simulink library "LibFactorGraph"  (Simulink 8.3)
settings: Solver=ode45  StartTime=0.0  StopTime=10.0  RelTol=1e-3
undefined symbols (not defined in the file or in its folder): bV, epsVal, eu, fcn, fP_0, fV, Hin_0, L_0, Nit_0, P_0, xi
libraries: LibFactorGraph x357
(part 1 of 4)
settings Model: Creator=amedeobuonanno  LastModifiedBy=amedeo.buonanno

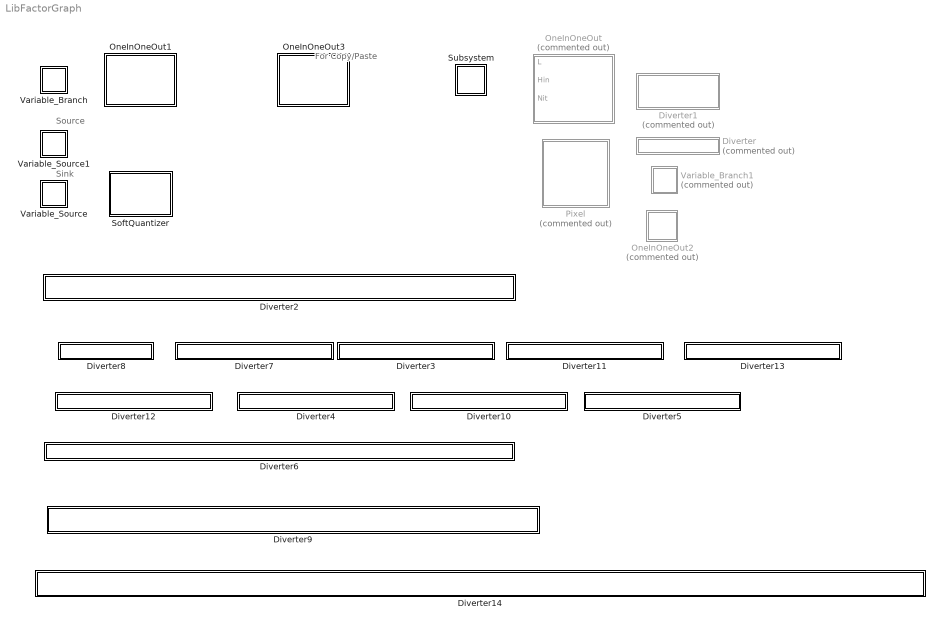
== system LibFactorGraph ==
  note: For Copy/Paste
  note: Source
  note: Sink
  Diverter : Subsystem  Commented=on  mask{up1=up1, up2=up2, down1=down1}
      mask prompts: up1 "Variable Up1"; up2 "Variable Up2"; down1 "Variable Down1"
      mask init:
      | % Set mask modifiable useful?
      | set_param(gcb,'MaskSelfModifiable','on');
      mask Display:
      | %port_label('lconn',1,up1);
      | %port_label('lconn',2,up2);
      | %port_label('rconn',1,down1);
  Diverter1 : Subsystem  Commented=on  mask{up1=up1, up2=up2, down1=down1}
      mask prompts: up1 "Variable Up1"; up2 "Variable Up2"; down1 "Variable Down1"
      mask init:
      | % Set mask modifiable useful?
      | set_param(gcb,'MaskSelfModifiable','on');
      mask Display:
      | port_label('lconn',1,up1);
      | port_label('lconn',2,up2);
      | port_label('rconn',1,down1);
  Diverter10 : Subsystem
      mask init:
      | % Set mask modifiable useful?
      | set_param(gcb,'MaskSelfModifiable','on');
  Diverter11 : Subsystem
      mask init:
      | % Set mask modifiable useful?
      | set_param(gcb,'MaskSelfModifiable','on');
  Diverter12 : Subsystem
      mask init:
      | % Set mask modifiable useful?
      | set_param(gcb,'MaskSelfModifiable','on');
  Diverter13 : Subsystem
      mask init:
      | % Set mask modifiable useful?
      | set_param(gcb,'MaskSelfModifiable','on');
  Diverter14 : Subsystem
      mask init:
      | % Set mask modifiable useful?
      | set_param(gcb,'MaskSelfModifiable','on');
  Diverter2 : Subsystem
      mask init:
      | % Set mask modifiable useful?
      | set_param(gcb,'MaskSelfModifiable','on');
  Diverter3 : Subsystem
      mask init:
      | % Set mask modifiable useful?
      | set_param(gcb,'MaskSelfModifiable','on');
  Diverter4 : Subsystem
      mask init:
      | % Set mask modifiable useful?
      | set_param(gcb,'MaskSelfModifiable','on');
  Diverter5 : Subsystem
      mask init:
      | % Set mask modifiable useful?
      | set_param(gcb,'MaskSelfModifiable','on');
  Diverter6 : Subsystem
      mask init:
      | % Set mask modifiable useful?
      | set_param(gcb,'MaskSelfModifiable','on');
  Diverter7 : Subsystem
      mask init:
      | % Set mask modifiable useful?
      | set_param(gcb,'MaskSelfModifiable','on');
  Diverter8 : Subsystem
      mask init:
      | % Set mask modifiable useful?
      | set_param(gcb,'MaskSelfModifiable','on');
  Diverter9 : Subsystem
      mask init:
      | % Set mask modifiable useful?
      | set_param(gcb,'MaskSelfModifiable','on');
  OneInOneOut : Subsystem  Commented=on  mask{L=0, Hin=0, Nit=0}
      mask prompts: L "Learning Mask"; Hin "Initial Matrix"; Nit "Iterations"
  OneInOneOut1 : Subsystem  mask{var=0}
      mask prompts: var "Name"
      mask init:
      | % Set mask modifiable useful?
      | set_param(gcb,'MaskSelfModifiable','on');
      | 
      | %Handles of the workspaces block to rename
      | set_param([gcb '/Constant'],'value', strcat('L_',var));
      | set_param([gcb '/Constant1'],'value', strcat('Hin_',var));
      | set_param([gcb '/Constant2'],'value', strcat('Nit_',var));
      | 
      | set_param([gcb '/To Workspace'],'variablename', strcat('H_',var));
      settings: CopyFcn=|
      | tmp = get_param([gcb '/To Workspace'],'variablename');
      | disp(tmp)
      | set_param([gcb '/To Workspace'],'variablename', strcat(tmp,'BOH'));
      mask Display:
      | fprintf(['P(Y|X)-' var]);
      | 
      | port_label('lconn',1,'Y');
      | port_label('rconn',1,'X');
  OneInOneOut2 : Subsystem  Commented=on  mask{var=0}
      mask prompts: var "Name"
      mask init:
      | % Set mask modifiable useful?
      | set_param(gcb,'MaskSelfModifiable','on');
      | 
      | %Handles of the workspaces block to rename
      | set_param([gcb '/Constant'],'value', strcat('fP_',var));
      | set_param([gcb '/Constant1'],'value', strcat('P_',var));
      | set_param([gcb '/Constant2'],'value', strcat('L_',var));
      | 
      | %set_param([gcb '/To Workspace'],'variablename', strcat('_',var));
      mask Display:
      | fprintf(['P-' var]);
      | 
      | %port_label('rconn',1,'X');
  OneInOneOut3 : Subsystem  Description=Permette la copia incolla di uno stesso blocco modificando solo il ToWorkspace  mask{var=0}
      mask prompts: var "Name"
      mask init:
      | % Set mask modifiable useful?
      | set_param(gcb,'MaskSelfModifiable','on');
      | 
      | %Handles of the workspaces block to rename
      | set_param([gcb '/Constant'],'value', strcat('L_',var));
      | set_param([gcb '/Constant1'],'value', strcat('Hin_',var));
      | set_param([gcb '/Constant2'],'value', strcat('Nit_',var));
      | 
      | set_param([gcb '/To Workspace'],'variablename', strcat('H_',num2str(randi(1000)),'_',num2str(randi(1000))));
      settings: CopyFcn=|
      | tmp = get_param([gcb '/To Workspace'],'variablename');
      | 
      | set_param([gcb '/To Workspace'],'variablename', strcat(tmp, num2str(randi(100))));
      mask Display:
      | fprintf(['P(Y|X)-' var]);
      | 
      | port_label('lconn',1,'Y');
      | port_label('rconn',1,'X');
  Pixel : Subsystem  Commented=on
  SoftQuantizer : Subsystem
      mask Display:
      | fprintf('Q');
      | 
      | port_label('lconn',1,'Xq');
      | port_label('rconn',1,'Xa');
  Subsystem : Subsystem
  Variable_Branch : Subsystem  mask{var=V}
      mask prompts: var "Variable"
      mask init:
      | % Set mask modifiable useful?
      | set_param(gcb,'MaskSelfModifiable','on');
      | 
      | %Handles of the workspaces block to rename
      | set_param([gcb '/To Workspace'],'variablename', strcat('f',var));
      | set_param([gcb '/To Workspace1'],'variablename', strcat('b',var));
      mask Display:
      | fprintf([var]);
      | 
      | port_label('lconn',1,'|');
      | port_label('rconn',1,'-');
      | 
      | t = 0:pi/6:2*pi;
      | plot(cos(t), sin(t))
  Variable_Branch1 : Subsystem  Commented=on  mask{var=V}
      mask prompts: var "Variable"
      mask init:
      | % Set mask modifiable useful?
      | set_param(gcb,'MaskSelfModifiable','on');
      mask Display:
      | fprintf([var]);
      | 
      | port_label('lconn',1,'|');
      | port_label('rconn',1,'-');
  Variable_Source : Subsystem  mask{var=V}
      mask prompts: var "Variable"
      mask init:
      | % Set mask modifiable useful?
      | set_param(gcb,'MaskSelfModifiable','on');
      | 
      | %Handles of the workspaces block to rename
      | set_param([gcb '/To Workspace'],'variablename', strcat('f',var));
      | set_param([gcb '/Constant'],'value', strcat('b',var));
      mask Display:
      | fprintf(var);
      | 
      | t = 0:pi/6:2*pi;
      | plot(cos(t), sin(t))
  Variable_Source1 : Subsystem  mask{var=V}
      mask prompts: var "Variable"
      mask init:
      | % Set mask modifiable useful?
      | set_param(gcb,'MaskSelfModifiable','on');
      | 
      | %Handles of the workspaces block to rename
      | set_param([gcb '/To Workspace'],'variablename', strcat('b',var));
      | set_param([gcb '/Constant'],'value', strcat('f',var));
      mask Display:
      | fprintf(var);
      | 
      | t = 0:pi/6:2*pi;
      | plot(cos(t), sin(t))

== system LibFactorGraph/Diverter ==
  Interpreted MATLAB Function : MATLABFcn  MATLABFcn=fcn(u)  Output1D=off
  Interpreted MATLAB Function1 : MATLABFcn  MATLABFcn=fcn(u)  Output1D=off
  Interpreted MATLAB Function2 : MATLABFcn  MATLABFcn=fcn(u)  Output1D=off
  Memory : Memory
  Memory1 : Memory
  Memory2 : Memory
  Product1 : Product  RndMeth=Zero
  Product2 : Product  RndMeth=Zero
  Product3 : Product  RndMeth=Zero
  Two-Way Connection1 : TwoWayConnection
  Two-Way Connection2 : TwoWayConnection
  Two-Way Connection5 : TwoWayConnection
  f_b_up1 : PMIOPort  Port=1  Side=Left
  f_b_up2 : PMIOPort  Port=2  Side=Left
  f_b_down1 : PMIOPort  Port=3  Side=Right
  wires:
  Product2/1 -> Interpreted MATLAB Function2/1
  Product1/1 -> Interpreted MATLAB Function1/1
  Product3/1 -> Interpreted MATLAB Function/1
  Two-Way Connection2/1 -> Memory/1
  Two-Way Connection1/1 -> Memory1/1
  Interpreted MATLAB Function/1 -> Two-Way Connection2/1
  Interpreted MATLAB Function1/1 -> Two-Way Connection1/1
  Interpreted MATLAB Function2/1 -> Two-Way Connection5/1
  Memory/1 -> Product1/1, Product2/1
  Memory1/1 -> Product3/2, Product2/2
  Two-Way Connection5/1 -> Memory2/1
  Memory2/1 -> Product1/2, Product3/1
  connections:
  f_b_up1/RConn1 -- Two-Way Connection2/RConn1
  f_b_up2/RConn1 -- Two-Way Connection1/RConn1
  f_b_down1/RConn1 -- Two-Way Connection5/RConn1

== system LibFactorGraph/Diverter1 ==
  Interpreted MATLAB Function : MATLABFcn  MATLABFcn=fcn(u)  Output1D=off
  Interpreted MATLAB Function1 : MATLABFcn  MATLABFcn=fcn(u)  Output1D=off
  Interpreted MATLAB Function2 : MATLABFcn  MATLABFcn=fcn(u)  Output1D=off
  Product1 : Product  RndMeth=Zero
  Product2 : Product  RndMeth=Zero
  Product3 : Product  RndMeth=Zero
  Two-Way Connection1 : TwoWayConnection
  Two-Way Connection2 : TwoWayConnection
  Two-Way Connection5 : TwoWayConnection
  f_b_up1 : PMIOPort  Port=1  Side=Left
  f_b_up2 : PMIOPort  Port=2  Side=Left
  f_b_down1 : PMIOPort  Port=3  Side=Right
  wires:
  Interpreted MATLAB Function2/1 -> Two-Way Connection5/1
  Interpreted MATLAB Function1/1 -> Two-Way Connection1/1
  Interpreted MATLAB Function/1 -> Two-Way Connection2/1
  Two-Way Connection1/1 -> Product2/2, Product3/2
  Two-Way Connection2/1 -> Product2/1, Product1/1
  Product3/1 -> Interpreted MATLAB Function/1
  Product1/1 -> Interpreted MATLAB Function1/1
  Two-Way Connection5/1 -> Product3/1, Product1/2
  Product2/1 -> Interpreted MATLAB Function2/1
  connections:
  f_b_down1/RConn1 -- Two-Way Connection5/RConn1
  f_b_up2/RConn1 -- Two-Way Connection1/RConn1
  f_b_up1/RConn1 -- Two-Way Connection2/RConn1

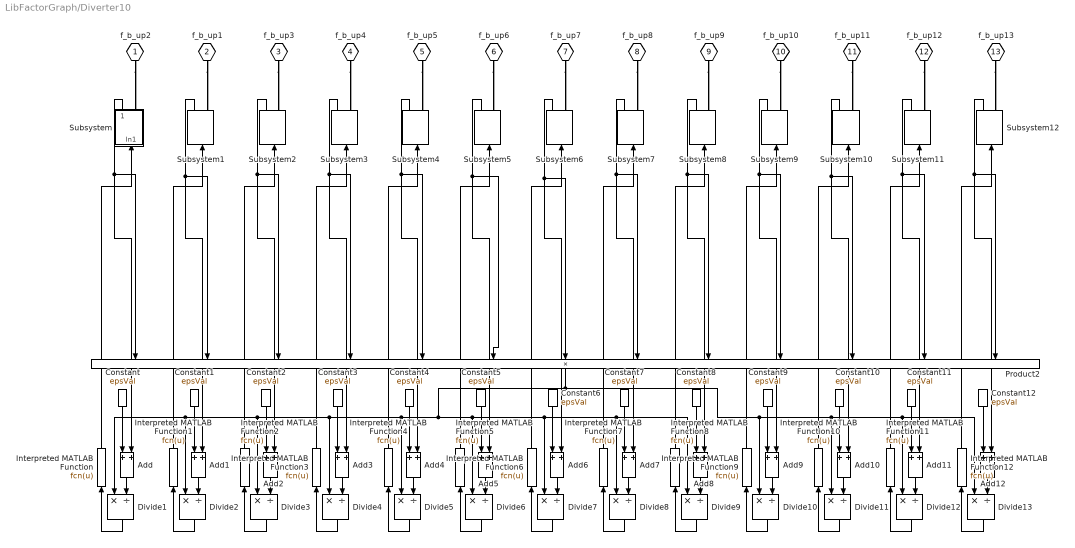
== system LibFactorGraph/Diverter10 ==
  Add{,1..12} (13 alike) : Sum
  Constant{,1..12} (13 alike) : Constant  Value=epsVal
  Divide{1..13} (13 alike) : Product  Inputs=*/
  Interpreted MATLAB Function{,1..12} (13 alike) : MATLABFcn  MATLABFcn=fcn(u)  Output1D=off
  Product2 : Product  Inputs=13  RndMeth=Zero
  Subsystem : Subsystem
  Subsystem{1..3,5..8,10..12} (10 alike) : LibFactorGraph/Diverter3/Subsystem
  Subsystem4 : LibFactorGraph/Diverter4/Subsystem
  Subsystem9 : LibFactorGraph/Diverter5/Subsystem
  f_b_up2 : PMIOPort  Port=1  Side=Left
  f_b_up1 : PMIOPort  Port=2  Side=Right
  f_b_up3 : PMIOPort  Port=3  Side=Left
  f_b_up4 : PMIOPort  Port=4  Side=Right
  f_b_up5 : PMIOPort  Port=5  Side=Left
  f_b_up6 : PMIOPort  Port=6  Side=Right
  f_b_up7 : PMIOPort  Port=7  Side=Left
  f_b_up8 : PMIOPort  Port=8  Side=Right
  f_b_up9 : PMIOPort  Port=9  Side=Left
  f_b_up10 : PMIOPort  Port=10  Side=Right
  f_b_up11 : PMIOPort  Port=11  Side=Left
  f_b_up12 : PMIOPort  Port=12  Side=Right
  f_b_up13 : PMIOPort  Port=13  Side=Left
  wires:
  Divide4/1 -> Interpreted MATLAB Function3/1
  Subsystem3/1 -> Add3/2, Product2/4
  Interpreted MATLAB Function3/1 -> Subsystem3/1
  Add3/1 -> Divide4/2
  Constant3/1 -> Add3/1
  Divide3/1 -> Interpreted MATLAB Function2/1
  Subsystem2/1 -> Add2/2, Product2/3
  Interpreted MATLAB Function2/1 -> Subsystem2/1
  Add2/1 -> Divide3/2
  Constant2/1 -> Add2/1
  Divide2/1 -> Interpreted MATLAB Function1/1
  Subsystem1/1 -> Product2/2, Add1/2
  Interpreted MATLAB Function1/1 -> Subsystem1/1
  Add1/1 -> Divide2/2
  Constant1/1 -> Add1/1
  Divide1/1 -> Interpreted MATLAB Function/1
  Subsystem/1(Out1) -> Product2/1, Add/2
  Interpreted MATLAB Function/1 -> Subsystem/1(In1)
  Add/1 -> Divide1/2
  Constant/1 -> Add/1
  Divide8/1 -> Interpreted MATLAB Function7/1
  Subsystem7/1 -> Product2/8, Add7/2
  Interpreted MATLAB Function7/1 -> Subsystem7/1
  Add7/1 -> Divide8/2
  Constant7/1 -> Add7/1
  Divide7/1 -> Interpreted MATLAB Function6/1
  Subsystem6/1 -> Product2/7, Add6/2
  Interpreted MATLAB Function6/1 -> Subsystem6/1
  Add6/1 -> Divide7/2
  Constant6/1 -> Add6/1
  Divide6/1 -> Interpreted MATLAB Function5/1
  Subsystem5/1 -> Product2/6, Add5/2
  Interpreted MATLAB Function5/1 -> Subsystem5/1
  Add5/1 -> Divide6/2
  Constant5/1 -> Add5/1
  Divide5/1 -> Interpreted MATLAB Function4/1
  Subsystem4/1 -> Product2/5, Add4/2
  Interpreted MATLAB Function4/1 -> Subsystem4/1
  Add4/1 -> Divide5/2
  Constant4/1 -> Add4/1
  Divide9/1 -> Interpreted MATLAB Function8/1
  Subsystem8/1 -> Product2/9, Add8/2
  Interpreted MATLAB Function8/1 -> Subsystem8/1
  Add8/1 -> Divide9/2
  Constant8/1 -> Add8/1
  Divide13/1 -> Interpreted MATLAB Function12/1
  Subsystem12/1 -> Product2/13, Add12/2
  Interpreted MATLAB Function12/1 -> Subsystem12/1
  Add12/1 -> Divide13/2
  Constant12/1 -> Add12/1
  Divide12/1 -> Interpreted MATLAB Function11/1
  Subsystem11/1 -> Product2/12, Add11/2
  Interpreted MATLAB Function11/1 -> Subsystem11/1
  Add11/1 -> Divide12/2
  Constant11/1 -> Add11/1
  Divide11/1 -> Interpreted MATLAB Function10/1
  Subsystem10/1 -> Product2/11, Add10/2
  Interpreted MATLAB Function10/1 -> Subsystem10/1
  Add10/1 -> Divide11/2
  Constant10/1 -> Add10/1
  Divide10/1 -> Interpreted MATLAB Function9/1
  Subsystem9/1 -> Product2/10, Add9/2
  Interpreted MATLAB Function9/1 -> Subsystem9/1
  Add9/1 -> Divide10/2
  Constant9/1 -> Add9/1
  Product2/1 -> Divide13/1, Divide12/1, Divide11/1, Divide10/1, Divide5/1, Divide1/1, Divide2/1, Divide3/1, Divide4/1, Divide9/1, Divide8/1, Divide7/1, Divide6/1
  connections:
  f_b_up4/RConn1 -- Subsystem3/RConn1
  f_b_up3/RConn1 -- Subsystem2/RConn1
  f_b_up1/RConn1 -- Subsystem1/RConn1
  f_b_up2/RConn1 -- Subsystem/RConn1
  f_b_up5/RConn1 -- Subsystem4/RConn1
  f_b_up6/RConn1 -- Subsystem5/RConn1
  f_b_up8/RConn1 -- Subsystem7/RConn1
  f_b_up7/RConn1 -- Subsystem6/RConn1
  f_b_up9/RConn1 -- Subsystem8/RConn1
  f_b_up10/RConn1 -- Subsystem9/RConn1
  f_b_up11/RConn1 -- Subsystem10/RConn1
  f_b_up12/RConn1 -- Subsystem11/RConn1
  f_b_up13/RConn1 -- Subsystem12/RConn1

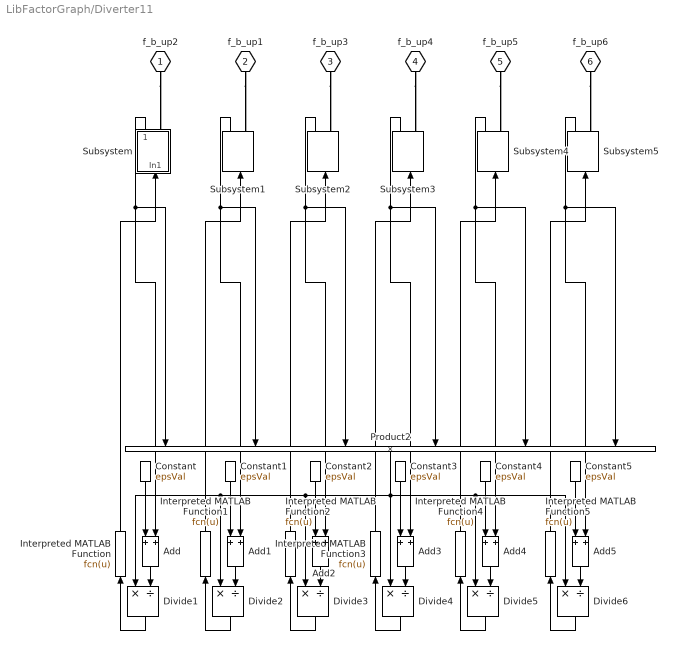
== system LibFactorGraph/Diverter11 ==
  Add{,1..5} (6 alike) : Sum
  Constant{,1..5} (6 alike) : Constant  Value=epsVal
  Divide{1..6} (6 alike) : Product  Inputs=*/
  Interpreted MATLAB Function{,1..5} (6 alike) : MATLABFcn  MATLABFcn=fcn(u)  Output1D=off
  Product2 : Product  Inputs=6  RndMeth=Zero
  Subsystem : Subsystem
  Subsystem{1..5} (5 alike) : LibFactorGraph/Diverter3/Subsystem
  f_b_up2 : PMIOPort  Port=1  Side=Left
  f_b_up1 : PMIOPort  Port=2  Side=Right
  f_b_up3 : PMIOPort  Port=3  Side=Left
  f_b_up4 : PMIOPort  Port=4  Side=Right
  f_b_up5 : PMIOPort  Port=5  Side=Left
  f_b_up6 : PMIOPort  Port=6  Side=Right
  wires:
  Divide5/1 -> Interpreted MATLAB Function4/1
  Subsystem4/1 -> Add4/2, Product2/5
  Interpreted MATLAB Function4/1 -> Subsystem4/1
  Add4/1 -> Divide5/2
  Constant4/1 -> Add4/1
  Divide4/1 -> Interpreted MATLAB Function3/1
  Subsystem3/1 -> Add3/2, Product2/4
  Interpreted MATLAB Function3/1 -> Subsystem3/1
  Add3/1 -> Divide4/2
  Constant3/1 -> Add3/1
  Divide3/1 -> Interpreted MATLAB Function2/1
  Subsystem2/1 -> Add2/2, Product2/3
  Interpreted MATLAB Function2/1 -> Subsystem2/1
  Add2/1 -> Divide3/2
  Constant2/1 -> Add2/1
  Divide2/1 -> Interpreted MATLAB Function1/1
  Subsystem1/1 -> Add1/2, Product2/2
  Interpreted MATLAB Function1/1 -> Subsystem1/1
  Add1/1 -> Divide2/2
  Constant1/1 -> Add1/1
  Divide1/1 -> Interpreted MATLAB Function/1
  Subsystem/1(Out1) -> Product2/1, Add/2
  Interpreted MATLAB Function/1 -> Subsystem/1(In1)
  Add/1 -> Divide1/2
  Constant/1 -> Add/1
  Divide6/1 -> Interpreted MATLAB Function5/1
  Subsystem5/1 -> Product2/6, Add5/2
  Interpreted MATLAB Function5/1 -> Subsystem5/1
  Add5/1 -> Divide6/2
  Constant5/1 -> Add5/1
  Product2/1 -> Divide3/1, Divide1/1, Divide2/1, Divide4/1, Divide6/1, Divide5/1
  connections:
  f_b_up5/RConn1 -- Subsystem4/RConn1
  f_b_up4/RConn1 -- Subsystem3/RConn1
  f_b_up3/RConn1 -- Subsystem2/RConn1
  f_b_up1/RConn1 -- Subsystem1/RConn1
  f_b_up2/RConn1 -- Subsystem/RConn1
  f_b_up6/RConn1 -- Subsystem5/RConn1

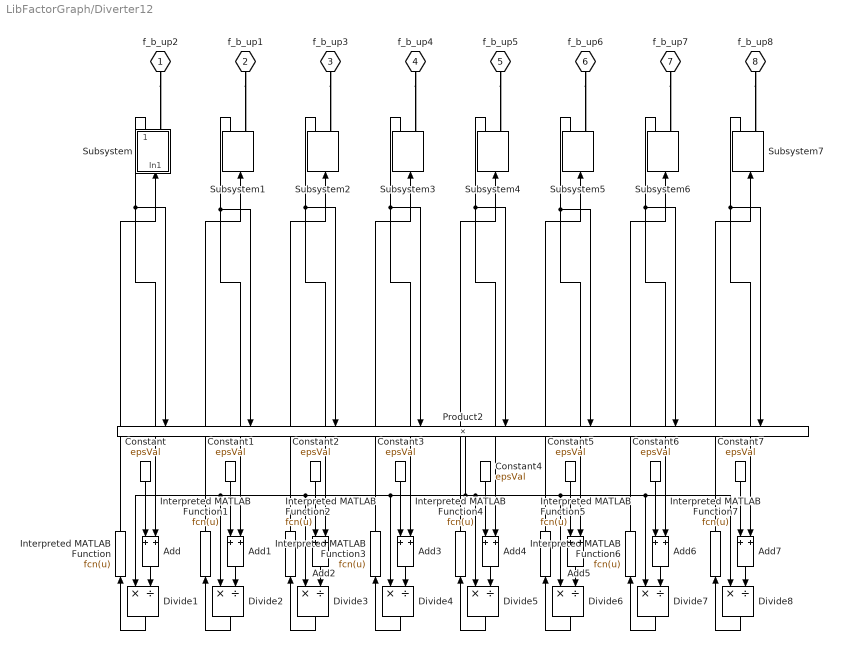
== system LibFactorGraph/Diverter12 ==
  Add{,1..7} (8 alike) : Sum
  Constant{,1..7} (8 alike) : Constant  Value=epsVal
  Divide{1..8} (8 alike) : Product  Inputs=*/
  Interpreted MATLAB Function{,1..7} (8 alike) : MATLABFcn  MATLABFcn=fcn(u)  Output1D=off
  Product2 : Product  Inputs=8  RndMeth=Zero
  Subsystem : Subsystem
  Subsystem{1..3,5..7} (6 alike) : LibFactorGraph/Diverter3/Subsystem
  Subsystem4 : LibFactorGraph/Diverter4/Subsystem
  f_b_up2 : PMIOPort  Port=1  Side=Left
  f_b_up1 : PMIOPort  Port=2  Side=Right
  f_b_up3 : PMIOPort  Port=3  Side=Left
  f_b_up4 : PMIOPort  Port=4  Side=Right
  f_b_up5 : PMIOPort  Port=5  Side=Left
  f_b_up6 : PMIOPort  Port=6  Side=Right
  f_b_up7 : PMIOPort  Port=7  Side=Left
  f_b_up8 : PMIOPort  Port=8  Side=Right
  wires:
  Divide4/1 -> Interpreted MATLAB Function3/1
  Subsystem3/1 -> Add3/2, Product2/4
  Interpreted MATLAB Function3/1 -> Subsystem3/1
  Add3/1 -> Divide4/2
  Constant3/1 -> Add3/1
  Divide3/1 -> Interpreted MATLAB Function2/1
  Subsystem2/1 -> Add2/2, Product2/3
  Interpreted MATLAB Function2/1 -> Subsystem2/1
  Add2/1 -> Divide3/2
  Constant2/1 -> Add2/1
  Divide2/1 -> Interpreted MATLAB Function1/1
  Subsystem1/1 -> Product2/2, Add1/2
  Interpreted MATLAB Function1/1 -> Subsystem1/1
  Add1/1 -> Divide2/2
  Constant1/1 -> Add1/1
  Divide1/1 -> Interpreted MATLAB Function/1
  Subsystem/1(Out1) -> Product2/1, Add/2
  Interpreted MATLAB Function/1 -> Subsystem/1(In1)
  Add/1 -> Divide1/2
  Constant/1 -> Add/1
  Divide8/1 -> Interpreted MATLAB Function7/1
  Subsystem7/1 -> Product2/8, Add7/2
  Interpreted MATLAB Function7/1 -> Subsystem7/1
  Add7/1 -> Divide8/2
  Constant7/1 -> Add7/1
  Divide7/1 -> Interpreted MATLAB Function6/1
  Subsystem6/1 -> Product2/7, Add6/2
  Interpreted MATLAB Function6/1 -> Subsystem6/1
  Add6/1 -> Divide7/2
  Constant6/1 -> Add6/1
  Divide6/1 -> Interpreted MATLAB Function5/1
  Subsystem5/1 -> Product2/6, Add5/2
  Interpreted MATLAB Function5/1 -> Subsystem5/1
  Add5/1 -> Divide6/2
  Constant5/1 -> Add5/1
  Divide5/1 -> Interpreted MATLAB Function4/1
  Subsystem4/1 -> Product2/5, Add4/2
  Interpreted MATLAB Function4/1 -> Subsystem4/1
  Add4/1 -> Divide5/2
  Constant4/1 -> Add4/1
  Product2/1 -> Divide8/1, Divide7/1, Divide6/1, Divide5/1, Divide1/1, Divide2/1, Divide3/1, Divide4/1
  connections:
  f_b_up4/RConn1 -- Subsystem3/RConn1
  f_b_up3/RConn1 -- Subsystem2/RConn1
  f_b_up1/RConn1 -- Subsystem1/RConn1
  f_b_up2/RConn1 -- Subsystem/RConn1
  f_b_up5/RConn1 -- Subsystem4/RConn1
  f_b_up6/RConn1 -- Subsystem5/RConn1
  f_b_up8/RConn1 -- Subsystem7/RConn1
  f_b_up7/RConn1 -- Subsystem6/RConn1

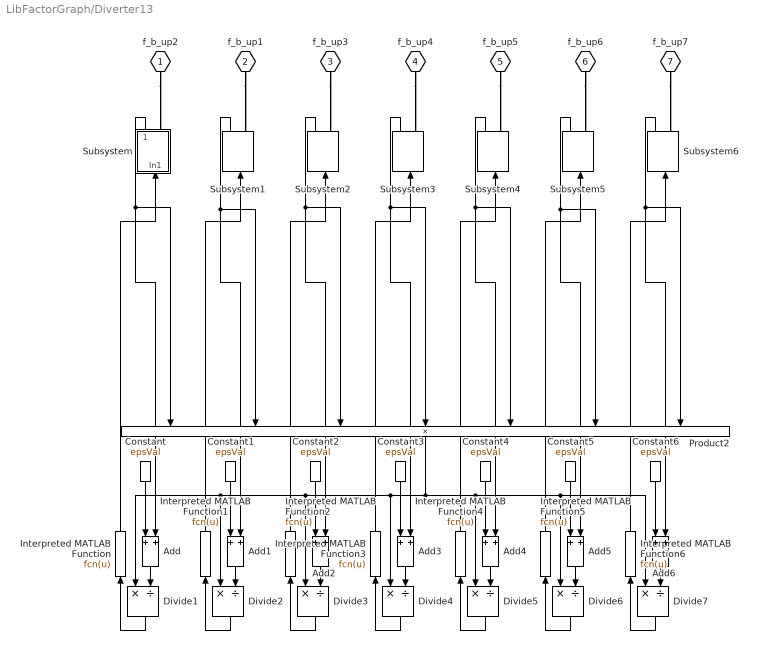
== system LibFactorGraph/Diverter13 ==
  Add{,1..6} (7 alike) : Sum
  Constant{,1..6} (7 alike) : Constant  Value=epsVal
  Divide{1..7} (7 alike) : Product  Inputs=*/
  Interpreted MATLAB Function{,1..6} (7 alike) : MATLABFcn  MATLABFcn=fcn(u)  Output1D=off
  Product2 : Product  Inputs=7  RndMeth=Zero
  Subsystem : Subsystem
  Subsystem{1..3,5..6} (5 alike) : LibFactorGraph/Diverter3/Subsystem
  Subsystem4 : LibFactorGraph/Diverter4/Subsystem
  f_b_up2 : PMIOPort  Port=1  Side=Left
  f_b_up1 : PMIOPort  Port=2  Side=Right
  f_b_up3 : PMIOPort  Port=3  Side=Left
  f_b_up4 : PMIOPort  Port=4  Side=Right
  f_b_up5 : PMIOPort  Port=5  Side=Left
  f_b_up6 : PMIOPort  Port=6  Side=Right
  f_b_up7 : PMIOPort  Port=7  Side=Left
  wires:
  Divide4/1 -> Interpreted MATLAB Function3/1
  Subsystem3/1 -> Add3/2, Product2/4
  Interpreted MATLAB Function3/1 -> Subsystem3/1
  Add3/1 -> Divide4/2
  Constant3/1 -> Add3/1
  Divide3/1 -> Interpreted MATLAB Function2/1
  Subsystem2/1 -> Add2/2, Product2/3
  Interpreted MATLAB Function2/1 -> Subsystem2/1
  Add2/1 -> Divide3/2
  Constant2/1 -> Add2/1
  Divide2/1 -> Interpreted MATLAB Function1/1
  Subsystem1/1 -> Product2/2, Add1/2
  Interpreted MATLAB Function1/1 -> Subsystem1/1
  Add1/1 -> Divide2/2
  Constant1/1 -> Add1/1
  Divide1/1 -> Interpreted MATLAB Function/1
  Subsystem/1(Out1) -> Product2/1, Add/2
  Interpreted MATLAB Function/1 -> Subsystem/1(In1)
  Add/1 -> Divide1/2
  Constant/1 -> Add/1
  Divide7/1 -> Interpreted MATLAB Function6/1
  Subsystem6/1 -> Product2/7, Add6/2
  Interpreted MATLAB Function6/1 -> Subsystem6/1
  Add6/1 -> Divide7/2
  Constant6/1 -> Add6/1
  Divide6/1 -> Interpreted MATLAB Function5/1
  Subsystem5/1 -> Product2/6, Add5/2
  Interpreted MATLAB Function5/1 -> Subsystem5/1
  Add5/1 -> Divide6/2
  Constant5/1 -> Add5/1
  Divide5/1 -> Interpreted MATLAB Function4/1
  Subsystem4/1 -> Product2/5, Add4/2
  Interpreted MATLAB Function4/1 -> Subsystem4/1
  Add4/1 -> Divide5/2
  Constant4/1 -> Add4/1
  Product2/1 -> Divide7/1, Divide6/1, Divide5/1, Divide1/1, Divide2/1, Divide3/1, Divide4/1
  connections:
  f_b_up4/RConn1 -- Subsystem3/RConn1
  f_b_up3/RConn1 -- Subsystem2/RConn1
  f_b_up1/RConn1 -- Subsystem1/RConn1
  f_b_up2/RConn1 -- Subsystem/RConn1
  f_b_up5/RConn1 -- Subsystem4/RConn1
  f_b_up6/RConn1 -- Subsystem5/RConn1
  f_b_up7/RConn1 -- Subsystem6/RConn1
